simulink model "kinetic_model"  (R2021b)
settings: Solver=VariableStepAuto  StartTime=0  StopTime=5631  FixedStep=1  RelTol=1e-5  AbsTol=1E-8
settings Model: Creator=castrove  LastModifiedBy=TonyZ
settings SolverCC: MaxOrder=2  AlgebraicLoopSolver=TrustRegion
settings DataIOCC: SaveFormat=Array  SignalLoggingSaveFormat=ModelDataLogs  SaveOutput=off  SaveTime=off  ReturnWorkspaceOutputs=off  SignalLoggingName=sigsOut  OutputTimes=2
settings OptimizationCC: BlockReduction=off  BooleanDataType=off
settings DebuggingCC: SaveWithParameterizedLinksMsg=none  UnderspecifiedInitializationDetection=Classic  MergeDetectMultiDrivingBlocksExec=none  SignalResolutionControl=TryResolveAllWithWarning  MultiTaskDSMMsg=warning  MultiTaskCondExecSysMsg=none  SFMachineParentedDataDiag=warning  ArithmeticOperatorsInVariantConditions=warning
settings HardwareCC: ProdBitPerPointer=32  ProdBitPerSizeT=32  ProdBitPerPtrDiffT=32  ProdLargestAtomicFloat=None  ProdIntDivRoundTo=Undefined  ProdEndianess=Unspecified  ProdWordSize=32  ProdHWDeviceType=32-bit Generic  TargetUnknown=on
settings ModelReferenceCC: PropagateSignalLabelsOutOfModel=off
settings SFSimCC: SimUseLocalCustomCode=off  CustomCodeUndefinedFunction=UseInterfaceOnly
settings RTWCC: TemplateMakefile=grt_unix.tmf  RTWUseLocalCustomCode=off
settings GRTTargetCC: TargetLangStandard=C89/C90 (ANSI)  CombineOutputUpdateFcns=off  GRTInterface=on
settings ConfigComp: CovMetricSettings=dw  CovSaveCumulativeToWorkspaceVar=on  CovSaveSingleToWorkspaceVar=on  CovExternalEMLEnable=off

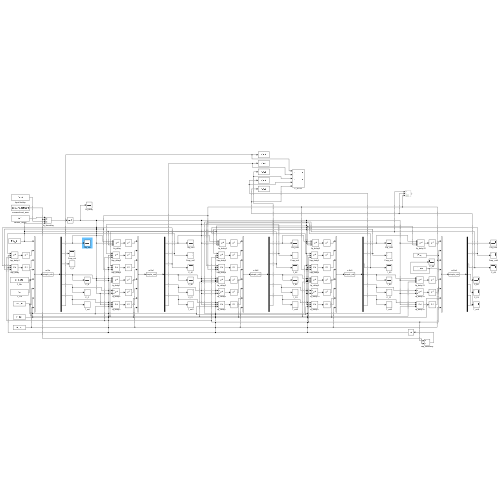
[thumbnail: Simulink's stored preview of the top-level diagram]
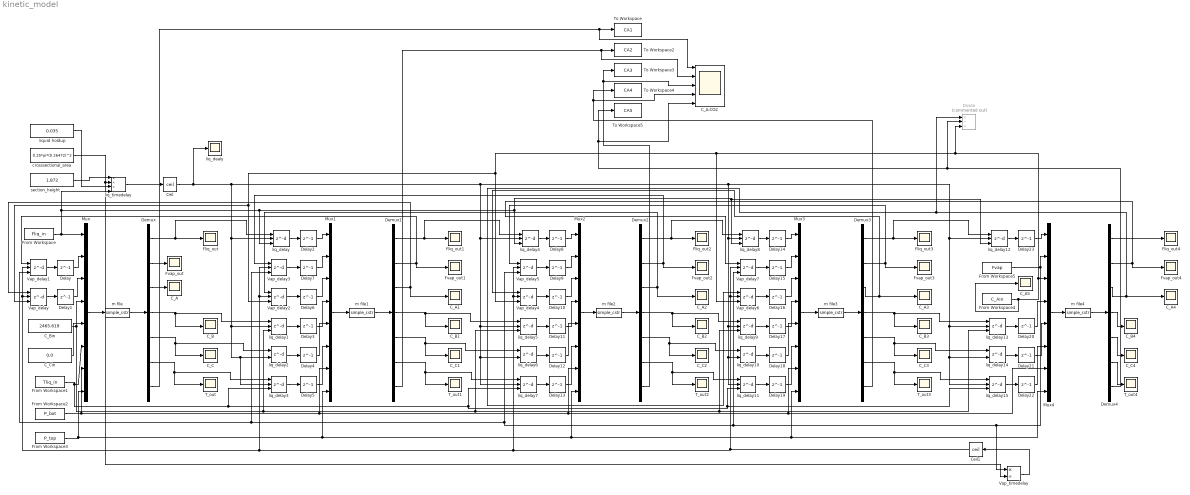
== system kinetic_model ==
  C_A{,1..5} (6 alike) : Scope
  C_A:CO2 : Scope  NumInputPorts=5
  C_B{,1..4} (5 alike) : Scope
  C_Bin : Constant  Value=2465.619
  C_C{,1..4} (5 alike) : Scope
  C_Cin : Constant  Value=0.0
  Ceil : Rounding  Operator=ceil
  Ceil1 : Rounding  Operator=ceil
  Delay{,1..23} (24 alike) : Delay  DelayLength=1  InitialCondition=0
  Demux{,1..4} (5 alike) : Demux  Outputs=7
      settings: DisplayOption=none
  Divide : Product  Commented=on  Inputs=*/*
  Fliq_out{,1..4} (5 alike) : Scope
  From Workspace : FromWorkspace  VariableName=Fliq_in  SampleTime=43  OutputAfterFinalValue=Holding final value
  From Workspace1 : FromWorkspace  VariableName=Tliq_in  SampleTime=43  OutputAfterFinalValue=Holding final value
  From Workspace2 : FromWorkspace  VariableName=P_bot  SampleTime=43  OutputAfterFinalValue=Holding final value
  From Workspace3 : FromWorkspace  VariableName=P_top  SampleTime=43  OutputAfterFinalValue=Holding final value
  From Workspace4 : FromWorkspace  VariableName=C_Ain  SampleTime=43  OutputAfterFinalValue=Holding final value
  From Workspace5 : FromWorkspace  VariableName=Fvap  SampleTime=43  OutputAfterFinalValue=Holding final value
  Fvap_out{,1..4} (5 alike) : Scope
  Mux{,1..4} (5 alike) : Mux  Inputs=8
  T_out{,1..4} (5 alike) : Scope
  To Workspace : ToWorkspace  VariableName=CA1  SampleTime=1
      settings: Save2DSignal=2-D array (concatenate along first dimension)
  To Workspace2 : ToWorkspace  VariableName=CA2  SampleTime=1
      settings: Save2DSignal=2-D array (concatenate along first dimension)
  To Workspace3 : ToWorkspace  VariableName=CA3  SampleTime=1
      settings: Save2DSignal=2-D array (concatenate along first dimension)
  To Workspace4 : ToWorkspace  VariableName=CA4  SampleTime=1
      settings: Save2DSignal=2-D array (concatenate along first dimension)
  To Workspace5 : ToWorkspace  VariableName=CA5  SampleTime=1
      settings: Save2DSignal=2-D array (concatenate along first dimension)
  Vap_delay{,2,4,6} (4 alike) : Delay  DelayLengthSource=Input port  DelayLength=1  InitialConditionSource=Input port  InitialCondition=0
      settings: InputPortMap=u0,p1,p4
  Vap_delay{1,3,5,7} (4 alike) : Delay  DelayLengthSource=Input port  DelayLength=1  InitialConditionSource=Input port  InitialCondition=1
      settings: InputPortMap=u0,p1,p4
  Vap_timedelay : Product  Inputs=*/
  crosssectional_area : Constant  Value=0.25*pi*(0.26472)^2
  liq_dealy : Scope
  liq_delay{,1,4..5,8} (5 alike) : Delay  DelayLengthSource=Input port  DelayLength=1  InitialConditionSource=Input port  InitialCondition=1
      settings: InputPortMap=u0,p1,p4
  liq_delay{2,6,10,14} (4 alike) : Delay  DelayLengthSource=Input port  DelayLength=1  InitialCondition=0
      settings: InputPortMap=u0,p1
  liq_delay{3,7,11,15} (4 alike) : Delay  DelayLengthSource=Input port  DelayLength=1  DelayLengthUpperLimit=1000  InitialConditionSource=Input port  InitialCondition=298
      settings: InputPortMap=u0,p1,p4
  liq_delay12 : Delay  DelayLengthSource=Input port  DelayLength=1  DelayLengthUpperLimit=1000  InitialConditionSource=Input port  InitialCondition=0
      settings: InputPortMap=u0,p1,p4
  liq_delay13 : Delay  DelayLengthSource=Input port  DelayLength=1  InitialConditionSource=Input port  InitialCondition=0
      settings: InputPortMap=u0,p1,p4
  liq_delay9 : Delay  DelayLengthSource=Input port  DelayLength=1  InitialConditionSource=Input port  InitialCondition=0
      settings: InputPortMap=u0,p1,p4
  liq_timedelay : Product  Inputs=***/
  liquid holdup : Constant  Value=0.035
  m file{,1..4} (5 alike) : S-Function  FunctionName=simple_cstr  Parameters=[500.6;1;1005.5;4380;1;1263;],[7.005e-05;0.0075752;0;2465.619;0;309.2792;]  SFunctionDeploymentMode=off  EnableBusSupport=off
  section_height : Constant  Value=1.872
  wires:
  m file/1 -> Demux/1
  Demux/3 -> C_A/1
  Demux/5 -> C_C/1, liq_delay2/1
  Mux/1 -> m file/1
  Demux/4 -> C_B/1, liq_delay1/1
  From Workspace/1 -> liq_delay/3, liq_delay12/3, liq_delay8/3, liq_delay4/3, liq_timedelay/4, Mux/1
  Demux/2 -> Fvap_out/1
  From Workspace1/1 -> liq_delay15/3, liq_delay11/3, liq_delay7/3, liq_delay3/3, Mux/6
  Demux/1 -> liq_delay/1, Fliq_out/1
  C_Bin/1 -> liq_delay13/3, liq_delay9/3, liq_delay5/3, liq_delay1/3, Mux/4
  Demux/6 -> T_out/1, liq_delay3/1
  C_Cin/1 -> Mux/5
  m file1/1 -> Demux1/1
  Mux1/1 -> m file1/1
  liq_delay/1 -> Delay2/1
  crosssectional_area/1 -> Vap_timedelay/2, liq_timedelay/2
  Vap_delay/1 -> Delay1/1
  liq_delay1/1 -> Delay3/1
  liq_delay2/1 -> Delay4/1
  liq_delay3/1 -> Delay5/1
  Vap_delay1/1 -> Delay/1
  Vap_delay2/1 -> Delay6/1
  Vap_delay3/1 -> Delay7/1
  liq_delay5/1 -> Delay11/1
  liq_delay7/1 -> Delay13/1
  liq_delay6/1 -> Delay12/1
  Demux1/4 -> C_B1/1, liq_delay5/1
  Demux1/6 -> T_out1/1, liq_delay7/1
  Demux1/1 -> liq_delay4/1, Fliq_out1/1
  Vap_delay4/1 -> Delay10/1
  Demux1/5 -> C_C1/1, liq_delay6/1
  Mux2/1 -> m file2/1
  liq_delay4/1 -> Delay8/1
  Vap_delay5/1 -> Delay9/1
  Demux2/3 -> C_A2/1, Vap_delay2/1
  Demux2/2 -> Fvap_out2/1, Vap_delay3/1
  Demux2/1 -> liq_delay8/1, Fliq_out2/1
  Demux2/4 -> C_B2/1, liq_delay9/1
  Demux2/6 -> T_out2/1, liq_delay11/1
  Demux2/5 -> C_C2/1, liq_delay10/1
  m file2/1 -> Demux2/1
  From Workspace4/1 -> C_A5/1, Divide/3, Vap_delay6/3, Vap_delay/3, Vap_delay2/3, Vap_delay4/3, Mux4/3
  liq_delay12/1 -> Delay23/1
  liq_delay14/1 -> Delay21/1
  liq_delay15/1 -> Delay22/1
  liq_delay11/1 -> Delay19/1
  liq_delay10/1 -> Delay18/1
  Demux3/3 -> C_A3/1, Vap_delay4/1
  Demux3/2 -> Fvap_out3/1, Vap_delay5/1
  Demux3/1 -> liq_delay12/1, Fliq_out3/1
  Demux3/4 -> C_B3/1, liq_delay13/1
  Demux3/6 -> T_out3/1, liq_delay15/1
  m file4/1 -> Demux4/1
  liq_timedelay/1 -> Ceil/1
  Mux4/1 -> m file4/1
  Mux3/1 -> m file3/1
  Demux4/1 -> Fliq_out4/1
  Demux4/5 -> C_C4/1
  Demux4/6 -> T_out4/1
  Vap_delay6/1 -> Delay16/1
  Demux4/2 -> Fvap_out4/1, Vap_delay7/1
  liq_delay13/1 -> Delay20/1
  Demux4/4 -> C_B4/1
  Demux3/5 -> C_C3/1, liq_delay14/1
  From Workspace5/1 -> Vap_delay1/3, Vap_delay3/3, Vap_delay5/3, Vap_delay7/3, Vap_timedelay/1, Mux4/2
  liq_delay8/1 -> Delay14/1
  liq_delay9/1 -> Delay17/1
  Demux4/3 -> C_A4/1, Divide/1, Vap_delay6/1
  m file3/1 -> Demux3/1
  Vap_delay7/1 -> Delay15/1
  Vap_timedelay/1 -> Ceil1/1
  Ceil/1 -> liq_dealy/1, liq_delay3/2, liq_delay2/2, liq_delay1/2, liq_delay/2, liq_delay11/2, liq_delay10/2, liq_delay9/2, liq_delay8/2, liq_delay15/2, liq_delay14/2, liq_delay13/2, liq_delay12/2, liq_delay7/2, liq_delay6/2, liq_delay5/2, liq_delay4/2
  Ceil1/1 -> Vap_delay5/2, Vap_delay4/2, Vap_delay3/2, Vap_delay2/2, Vap_delay1/2, Vap_delay/2, Vap_delay6/2, Vap_delay7/2
  Demux1/2 -> Fvap_out1/1, Vap_delay1/1
  Demux1/3 -> C_A1/1, Vap_delay/1
  Delay2/1 -> Mux1/1
  Delay3/1 -> Mux1/4
  Delay4/1 -> Mux1/5
  Delay5/1 -> Mux1/6
  Delay6/1 -> Mux1/3
  Delay7/1 -> Mux1/2
  Delay8/1 -> Mux2/1
  Delay9/1 -> Mux2/2
  Delay10/1 -> Mux2/3
  Delay11/1 -> Mux2/4
  Delay12/1 -> Mux2/5
  Delay13/1 -> Mux2/6
  Delay14/1 -> Mux3/1
  Delay15/1 -> Mux3/2
  Delay16/1 -> Mux3/3
  Delay17/1 -> Mux3/4
  Delay18/1 -> Mux3/5
  Delay19/1 -> Mux3/6
  Delay20/1 -> Mux4/4
  Delay21/1 -> Mux4/5
  Delay22/1 -> Mux4/6
  Delay23/1 -> Mux4/1
  section_height/1 -> liq_timedelay/1
  Delay/1 -> Mux/2
  Delay1/1 -> Mux/3
  liquid holdup/1 -> liq_timedelay/3
  Demux/7 -> C_A:CO2/1, To Workspace/1
  Demux1/7 -> C_A:CO2/2, To Workspace2/1
  Demux2/7 -> To Workspace3/1, C_A:CO2/3
  Demux3/7 -> To Workspace4/1, C_A:CO2/4
  Demux4/7 -> Divide/2, To Workspace5/1, C_A:CO2/5
  From Workspace2/1 -> Mux4/7, Mux3/7, Mux2/7, Mux1/7, Mux/7
  From Workspace3/1 -> Mux2/8, Mux4/8, Mux3/8, Mux1/8, Mux/8
